simulink subsystem "calculate_fault_injected_pwm"  (R2024a)
settings: Solver=VariableStepAuto  StartTime=0.0  StopTime=10.0  RelTol=1e-3
settings Model: Creator=UASG  LastModifiedBy=user

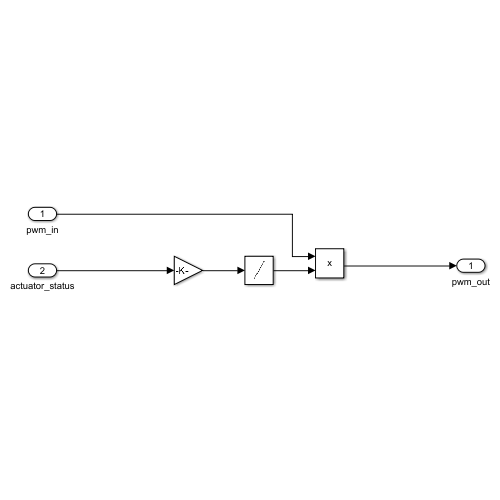
[thumbnail: Simulink's stored preview of the top-level diagram]
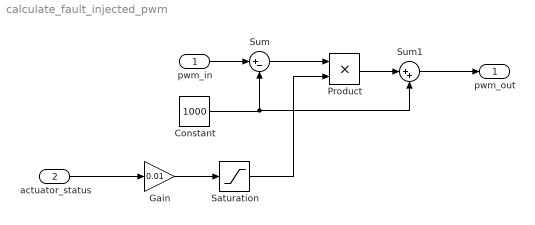
== system calculate_fault_injected_pwm ==
  pwm_in : Inport
  actuator_status : Inport  Port=2
  Constant : Constant  Value=1000  OutDataTypeStr=single
  Gain : Gain  Gain=0.01
  Product : Product
  Saturation : Saturate  UpperLimit=1  LowerLimit=0
  Sum : Sum  Inputs=|+-
  Sum1 : Sum  Inputs=|++
  pwm_out : Outport
  wires:
  actuator_status/1 -> Gain/1
  Gain/1 -> Saturation/1
  pwm_in/1 -> Sum/1
  Constant/1 -> Sum/2, Sum1/2
  Sum/1 -> Product/1
  Saturation/1 -> Product/2
  Product/1 -> Sum1/1
  Sum1/1 -> pwm_out/1
